simulink model "dspanc_fixpt_win32"  (Simulink 6.0)
settings: Solver=FixedStepDiscrete  StartTime=0.0  StopTime=inf  RelTol=1e-3
undefined symbols (not defined in the file or in its folder): wavread
libraries: simulink x4, dspsrcs4 x2, dspsnks4 x2, dsparch4 x1, dspsigops x1, dspadpt3 x1, dspwin32 x1
settings Model: Creator=navan  LastModifiedBy=mkhan  ExtModeAutoUpdateStatusClock=off
settings DataIOCC: LimitDataPoints=off  SaveOutput=off  SaveTime=off  SignalLoggingName=sigsOut
settings OptimizationCC: InlineInvariantSignals=off
settings DebuggingCC: CheckExecutionContextPreStartOutputMsg=on  CheckExecutionContextRuntimeOutputMsg=on  SolverPrmCheckMsg=none  IntegerOverflowMsg=none  ParameterPrecisionLossMsg=none
settings HardwareCC: TargetUnknown=on
settings ModelReferenceCC: UpdateModelReferenceTargets=IfOutOfDate
settings SFSimCC: SFSimApplyToAllLibs=on  SFSimBuildMode=Incremental

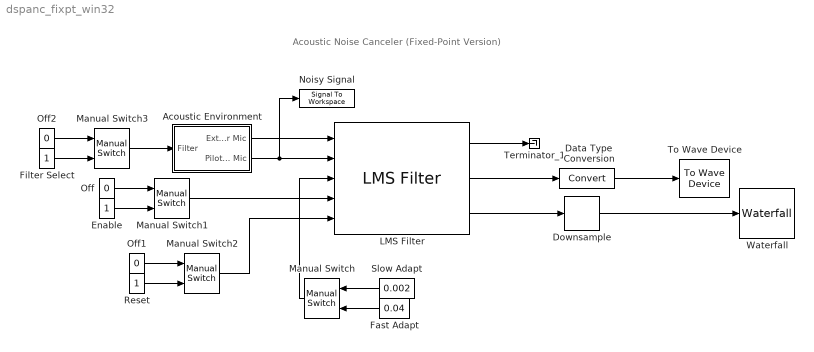
== system dspanc_fixpt_win32 ==
  note: Acoustic Noise Canceler (Fixed-Point Version)
  Acoustic Environment : Subsystem  PropExecContextAcrossSSBoundary=on
  Data Type  Conversion : DataTypeConversion  SaturateOnIntegerOverflow=on  RndMeth=Zero
  Downsample : dspsigops/Downsample  N=32  phase=0  ic=0  smode=Allow multirate  fmode=Maintain input frame size
  Enable : Constant  OutDataTypeMode=boolean
  Fast Adapt : Constant  Orientation=left  Value=0.04  OutDataTypeMode=Specify via dialog  OutScaling=2^-15
  Filter Select : Constant  OutDataTypeMode=boolean
  LMS Filter : dspadpt3/LMS Filter  DialogController=dspDDGCreate  DialogControllerArgs=DataTag1  Algo=Normalized LMS  L=40  stepflag=Input port  mu=0.1  leakage=1.0  ic=0  Adapt=on  resetflag=Non-zero sample  weights=on  firstCoeffMode=Binary point scaling  firstCoeffWordLength=16  firstCoeffFracLength=16  secondCoeffMode=User-defined  secondCoeffWordLength=2  secondCoeffFracLength=15  accumMode=Binary point scaling  accumWordLength=32  accumFracLength=20  accum2Mode=User-defined  accum2FracLength=20  prodOutputMode=Binary point scaling  prodOutputWordLength=32  prodOutputFracLength=20  memoryMode=Binary point scaling  memoryWordLength=16  memoryFracLength=15  roundingMode=Nearest  overflowMode=on  addnparflag=off
  Manual Switch : simulink/Signal Routing/Manual Switch  Orientation=left  sw=0  action=0
  Manual Switch1 : simulink/Signal Routing/Manual Switch  sw=0  action=0
  Manual Switch2 : simulink/Signal Routing/Manual Switch  sw=1  action=0
  Manual Switch3 : simulink/Signal Routing/Manual Switch  sw=1  action=0
  Noisy Signal : dspsnks4/Signal To Workspace  VariableName=y_noisy  FrameMode=Concatenate frames (2-D array)
      settings: FixptAsFi=off
  Off : Constant  Value=0  OutDataTypeMode=boolean
  Off1 : Constant  Value=0  OutDataTypeMode=boolean
  Off2 : Constant  Value=0  OutDataTypeMode=boolean
  Reset : Constant  OutDataTypeMode=boolean
  Slow Adapt : Constant  Orientation=left  Value=0.002  OutDataTypeMode=Specify via dialog  OutScaling=2^-15
  Terminator_1 : Terminator
  To Wave Device : dspwin32/To Wave Device  bufDuration=0.4  initDelay=0.05  useDefaultDevice=on  userDeviceID=Plantronics headset  enable24Bit=off
  Waterfall : dspsnks4/Waterfall  TraceProperties=off  NumTraces=6  CMapStr=autumn  TNewest=0.9  TOldest=0.5  HistoryLength=50  HistoryFull=Overwrite  UpdateInterval=1  ExportMode=All visible  MLExportName=ExportData  AutoExport=off  DisplayProperties=off  MouseMode=Orbit  AxisGrid=on  Snapshot=off  Suspend=off  SyncSnapshots=off  OpenScopeAtSimStart=off  FigPos=[27 57 405 339]  CameraView=[28.5695107359948 1316.8235109177 -294.350451091202 -0.004386576265097 22.5 3.5 0.594111941595966 -49.3321641526923 11.3523452384532 1.12783221137103 1 122.332173767783 16.310956502371]  InportDimsHint=[40 1]  AxisProperties=off  AxisColor='w'  XLabel=Amplitude  YLabel=Samples  ZLabel=Time  TriggerProperties=off  TrigStartMode=Immediately  TrigStartT=0  TrigStartN=0  TrigStartFcn=trigbegin  TrigStopMode=Never  TrigStopT=0.1  TrigStopN=1  TrigStopFcn=trigend  TrigRearmMode=Never  TrigRearmT=0  TrigRearmN=0  TrigRearmFcn=trigrearm  XformProperties=on  XformMode=None  XformFcn=abs  XformExpr=(u+1)/2
      settings: YMin=-0.188312025368214  YMax=0.17953887283802
  wires:
  Downsample/1 -> Waterfall/1
  Acoustic Environment/1(Exterior Mic) -> LMS Filter/1
  Slow Adapt/1 -> Manual Switch/1
  Fast Adapt/1 -> Manual Switch/2
  Manual Switch/1 -> LMS Filter/3
  LMS Filter/3 -> Downsample/1
  Acoustic Environment/2(Pilot's Mic) -> LMS Filter/2, Noisy Signal/1
  LMS Filter/2 -> Data Type  Conversion/1
  LMS Filter/1 -> Terminator_1/1
  Off/1 -> Manual Switch1/1
  Enable/1 -> Manual Switch1/2
  Off1/1 -> Manual Switch2/1
  Reset/1 -> Manual Switch2/2
  Manual Switch1/1 -> LMS Filter/4
  Manual Switch2/1 -> LMS Filter/5
  Off2/1 -> Manual Switch3/1
  Filter Select/1 -> Manual Switch3/2
  Manual Switch3/1 -> Acoustic Environment/1(Filter)
  Data Type  Conversion/1 -> To Wave Device/1

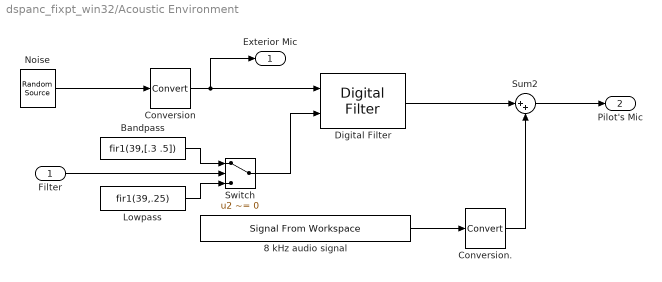
== system dspanc_fixpt_win32/Acoustic Environment ==
  Filter : Inport  LatchInput=off
  8 kHz audio signal : dspsrcs4/Signal From Workspace  X=int16((2^15)*(wavread('dspafxf_8000.wav')))  Ts=1/8000  nsamps=32  OutputAfterFinalValue=Cyclic repetition
  Bandpass : Constant  Value=fir1(39,[.3 .5])  OutDataTypeMode=Specify via dialog  OutScaling=2^-17
  Conversion : DataTypeConversion  OutDataTypeMode=Specify via dialog  OutScaling=2^-13  RndMeth=Nearest
  Conversion. : DataTypeConversion  OutDataTypeMode=Specify via dialog  OutScaling=2^-15  ConvertRealWorld=Stored Integer (SI)  RndMeth=Nearest
  Digital Filter : dsparch4/Digital Filter  DialogController=dspDDGCreate  DialogControllerArgs=DataTag0  TypePopup=FIR (all zeros)  IIRFiltStruct=Direct form II transposed  AllPoleFiltStruct=Direct form  FIRFiltStruct=Direct form  CoeffSource=Input port(s)  NumCoeffs=[1 2]  DenCoeffs=[1 0.1]  BiQuadCoeffs=[1 0.3 0.4 1 0.1 0.2]  LatticeCoeffs=[0.2 0.4]  denIgnore=on  FiltPerSampPopup=One filter per frame  IC=0  ICnum=0  ICden=0  accumMode=Binary point scaling  accumWordLength=32  accumFracLength=30  prodOutputMode=Binary point scaling  prodOutputWordLength=32  prodOutputFracLength=30  roundingMode=Nearest  overflowMode=off  ScaleValues=0  scaleValueFracLength=14  tapSumFracLength=30  stageInFracLength=15  stageOutFracLength=15
      settings: additionalParams=on  showOut=on  showAcc=on  showMpy=on
  Lowpass : Constant  Value=fir1(39,.25)  OutDataTypeMode=Specify via dialog  OutScaling=2^-17
  Noise : dspsrcs4/Random Source  SrcType=Gaussian  NormMethod=Sum of uniform values  CltLength=5  Min=-1  Max=1  Mean=0  Var=1  RepMode=Specify seed  Seed=[23341]  Inherit=off  SampMode=Discrete  SampTime=1/8000  SampFrame=32  DataType=Single  OutComplex=Real
  Sum2 : Sum  Inputs=|++  RndMeth=Nearest  SaturateOnIntegerOverflow=on
  Switch : Switch  Criteria=u2 ~= 0  SaturateOnIntegerOverflow=on
  Exterior Mic : Outport
  Pilot's Mic : Outport  Port=2
  wires:
  Noise/1 -> Conversion/1
  Conversion./1 -> Sum2/2
  Conversion/1 -> Exterior Mic/1, Digital Filter/1
  Lowpass/1 -> Switch/3
  Bandpass/1 -> Switch/1
  Switch/1 -> Digital Filter/2
  Digital Filter/1 -> Sum2/1
  Filter/1 -> Switch/2
  Sum2/1 -> Pilot's Mic/1
  8 kHz audio signal/1 -> Conversion./1
